simulink model "Trajectory_Tracking_Final"  (R2023b)
settings: Solver=ode1  StartTime=0.0  StopTime=100  FixedStep=SampleTime  MaxStep=0.01  RelTol=1e-3  EnableMultiTasking=on
values from neighbouring files (symbols this model uses):
  Delay = 3    [Prepare_MPC_005.m]
  FilterDer0 = [8.542800360484532896e-02 ... (first row only)    [Prepare_MPC_005.m]
  FilterDer1 = [2.939212680227305530e+00 ... (first row only)    [Prepare_MPC_005.m]
  SampleTime = 0.05    [Prepare_MPC_005.m]
undefined symbols (not defined in the file or in its folder): GetPosition, length_trajectory_s, poly_approx_trajectory, UpdateBoard, xx, yy
libraries: sldrtlib x1
(part 2 of 2)

== system Trajectory_Tracking_Final/Subsystem1/Subsystem/Subsystem5/Subsystem13 ==
  u : Inport
  MATLAB Function11 : MATLAB Function  TreatAsAtomicUnit=on
  MatrixMultiply : Product  Multiplication=Matrix(*)
  Out1 : Outport
  wires:
  [Filter_Coeff_1] -> MatrixMultiply/2
  MATLAB Function11/1(y) -> MatrixMultiply/1
  MatrixMultiply/1 -> Out1/1
  u/1 -> MATLAB Function11/1(u)
  [Initial_MAtrix_Buffer] -> MATLAB Function11/2(Initial_Buffer)

== system Trajectory_Tracking_Final/Subsystem1/Subsystem/Subsystem5/Subsystem14 ==
  u : Inport
  MATLAB Function11 : MATLAB Function  TreatAsAtomicUnit=on
  MatrixMultiply : Product  Multiplication=Matrix(*)
  Out1 : Outport
  wires:
  [Filter_Coeff_1] -> MatrixMultiply/2
  MATLAB Function11/1(y) -> MatrixMultiply/1
  MatrixMultiply/1 -> Out1/1
  u/1 -> MATLAB Function11/1(u)
  [Initial_MAtrix_Buffer] -> MATLAB Function11/2(Initial_Buffer)

== system Trajectory_Tracking_Final/Subsystem1/Subsystem/Subsystem5/Subsystem2 ==
  u : Inport
  MATLAB Function11 : MATLAB Function  TreatAsAtomicUnit=on
  MatrixMultiply : Product  Multiplication=Matrix(*)
  Out1 : Outport
  wires:
  [Filter_Coeff_0] -> MatrixMultiply/2
  MATLAB Function11/1(y) -> MatrixMultiply/1
  MatrixMultiply/1 -> Out1/1
  u/1 -> MATLAB Function11/1(u)
  [Initial_MAtrix_Buffer] -> MATLAB Function11/2(Initial_Buffer)

== system Trajectory_Tracking_Final/Subsystem1/Subsystem/Subsystem5/Subsystem3 ==
  u : Inport
  MATLAB Function11 : MATLAB Function  TreatAsAtomicUnit=on
  MatrixMultiply : Product  Multiplication=Matrix(*)
  Out1 : Outport
  wires:
  [Filter_Coeff_0] -> MatrixMultiply/2
  MATLAB Function11/1(y) -> MatrixMultiply/1
  MatrixMultiply/1 -> Out1/1
  u/1 -> MATLAB Function11/1(u)
  [Initial_MAtrix_Buffer] -> MATLAB Function11/2(Initial_Buffer)

== system Trajectory_Tracking_Final/Subsystem1/Subsystem/Subsystem5/Subsystem4 ==
  u : Inport
  MATLAB Function11 : MATLAB Function  TreatAsAtomicUnit=on
  MatrixMultiply : Product  Multiplication=Matrix(*)
  Out1 : Outport
  wires:
  [Filter_Coeff_0] -> MatrixMultiply/2
  MATLAB Function11/1(y) -> MatrixMultiply/1
  MatrixMultiply/1 -> Out1/1
  u/1 -> MATLAB Function11/1(u)
  [Initial_MAtrix_Buffer] -> MATLAB Function11/2(Initial_Buffer)

== system Trajectory_Tracking_Final/Subsystem1/Subsystem/Subsystem5/Subsystem5 ==
  u : Inport
  Discrete Filter Coefficents : Constant  Value=|
      | [1.574208515729901059e+01
      | 1.586094721714563072e+01
      | -5.994995630757394833e-01
      | -9.191365250349250005e+00
      | -1.170290325508502960e+01
      | -9.922366987693955309e+00
      | -5.638009858585491862e+00
      | -6.380852781707303523e-01
      | 3.289153343139662233e+00
      | 4.355452594936194188e+00
      | 7.725590668082207291e-01
      | -2.327967186368518515e+00]'
  MATLAB Function11 : MATLAB Function  TreatAsAtomicUnit=on
  MatrixMultiply : Product  Multiplication=Matrix(*)
  X_Vel : Outport
  wires:
  Discrete Filter Coefficents/1 -> MatrixMultiply/2
  MATLAB Function11/1(y) -> MatrixMultiply/1
  MatrixMultiply/1 -> X_Vel/1
  u/1 -> MATLAB Function11/1(u)

== system Trajectory_Tracking_Final/Subsystem1/Subsystem/Subsystem5/Subsystem6 ==
  u : Inport
  Discrete Filter Coefficents : Constant  Value=|
      | [1.574208515729901059e+01
      | 1.586094721714563072e+01
      | -5.994995630757394833e-01
      | -9.191365250349250005e+00
      | -1.170290325508502960e+01
      | -9.922366987693955309e+00
      | -5.638009858585491862e+00
      | -6.380852781707303523e-01
      | 3.289153343139662233e+00
      | 4.355452594936194188e+00
      | 7.725590668082207291e-01
      | -2.327967186368518515e+00]'
  MATLAB Function11 : MATLAB Function  TreatAsAtomicUnit=on
  MatrixMultiply : Product  Multiplication=Matrix(*)
  X_Vel1 : Outport
  wires:
  Discrete Filter Coefficents/1 -> MatrixMultiply/2
  MATLAB Function11/1(y) -> MatrixMultiply/1
  MatrixMultiply/1 -> X_Vel1/1
  u/1 -> MATLAB Function11/1(u)

== system Trajectory_Tracking_Final/Subsystem1/Subsystem/Subsystem5/Subsystem7 ==
  u : Inport
  Derivative : Derivative
  Discrete Filter Coefficents : Constant  Value=|
      | [1.574208515729901059e+01
      | 1.586094721714563072e+01
      | -5.994995630757394833e-01
      | -9.191365250349250005e+00
      | -1.170290325508502960e+01
      | -9.922366987693955309e+00
      | -5.638009858585491862e+00
      | -6.380852781707303523e-01
      | 3.289153343139662233e+00
      | 4.355452594936194188e+00
      | 7.725590668082207291e-01
      | -2.327967186368518515e+00]'
  MATLAB Function11 : MATLAB Function  TreatAsAtomicUnit=on
  MatrixMultiply : Product  Multiplication=Matrix(*)
  Scope : Scope  NumInputPorts=2
  Out1 : Outport
  wires:
  Discrete Filter Coefficents/1 -> MatrixMultiply/2
  MATLAB Function11/1(y) -> MatrixMultiply/1
  MatrixMultiply/1 -> Scope/1, Out1/1
  u/1 -> Derivative/1, MATLAB Function11/1(u)
  Derivative/1 -> Scope/2

== system Trajectory_Tracking_Final/Subsystem1/Subsystem/Subsystem5/Subsystem8 ==
  u : Inport
  Discrete Filter Coefficents : Constant  Value=|
      | [1.574208515729901059e+01
      | 1.586094721714563072e+01
      | -5.994995630757394833e-01
      | -9.191365250349250005e+00
      | -1.170290325508502960e+01
      | -9.922366987693955309e+00
      | -5.638009858585491862e+00
      | -6.380852781707303523e-01
      | 3.289153343139662233e+00
      | 4.355452594936194188e+00
      | 7.725590668082207291e-01
      | -2.327967186368518515e+00]'
  MATLAB Function11 : MATLAB Function  TreatAsAtomicUnit=on
  MatrixMultiply : Product  Multiplication=Matrix(*)
  Out1 : Outport
  wires:
  Discrete Filter Coefficents/1 -> MatrixMultiply/2
  MATLAB Function11/1(y) -> MatrixMultiply/1
  MatrixMultiply/1 -> Out1/1
  u/1 -> MATLAB Function11/1(u)

== system Trajectory_Tracking_Final/Subsystem1/Subsystem/Subsystem5/Subsystem9 ==
  u : Inport
  Derivative : Derivative
  Discrete Filter Coefficents : Constant  Value=|
      | [1.574208515729901059e+01
      | 1.586094721714563072e+01
      | -5.994995630757394833e-01
      | -9.191365250349250005e+00
      | -1.170290325508502960e+01
      | -9.922366987693955309e+00
      | -5.638009858585491862e+00
      | -6.380852781707303523e-01
      | 3.289153343139662233e+00
      | 4.355452594936194188e+00
      | 7.725590668082207291e-01
      | -2.327967186368518515e+00]'
  MATLAB Function11 : MATLAB Function  TreatAsAtomicUnit=on
  MatrixMultiply : Product  Multiplication=Matrix(*)
  Scope : Scope  NumInputPorts=2
  Out1 : Outport
  wires:
  Discrete Filter Coefficents/1 -> MatrixMultiply/2
  MATLAB Function11/1(y) -> MatrixMultiply/1
  Derivative/1 -> Scope/2
  u/1 -> Derivative/1, MATLAB Function11/1(u)
  MatrixMultiply/1 -> Scope/1, Out1/1

== matlab function Trajectory_Tracking_Final/Subsystem1/Subsystem/Subsystem5/MATLAB Function ==
  data: Initial_MAtrix output
function Initial_MAtrix = Immutable_Constant_Matrix()

Initial_MAtrix = ones(10,1);

== matlab function Trajectory_Tracking_Final/Subsystem1/Subsystem/Limit Input/MATLAB Function5 ==
  data: PWL input; PWL_Limit output; Position input; epsilon input
function PWL_Limit = fcn(PWL,Position,epsilon)

if (PWL < 0) && (Position-epsilon <= 0)
 PWL_Limit = 0;
else if (PWL > 0) && (Position+epsilon >= 0.49876)
     PWL_Limit = 0    ;
else
 PWL_Limit = PWL;
end
end

== matlab function Trajectory_Tracking_Final/Subsystem1/Subsystem/Limit Input/MATLAB Function6 ==
  data: PWL input; PWL_Limit output; Position input; epsilon input

function PWL_Limit = fcn(PWL,Position,epsilon)

if (PWL < 0) && (Position-epsilon <= 0)
 PWL_Limit = 0;
else if (PWL > 0) && (Position+epsilon >= 0.62159)
     PWL_Limit = 0    ;
else
 PWL_Limit = PWL;
end
end

== matlab function Trajectory_Tracking_Final/SOLVE OCP /Subsystem/Delete L ==
  data: x10 input; x_8 output
function x_8 = fcn(x10)
relevantstates = [1,2,4,5,6,7,9,10];
x_8 =x10(relevantstates);

== matlab function Trajectory_Tracking_Final/SOLVE OCP /Subsystem5/MPC 1/MATLAB Function ==
  data: x input; x_warm output
function x_warm = fcn(x)
x_warm = [x(:,3:end) x(:,end)];

== matlab function Trajectory_Tracking_Final/Subsystem1/Subsystem/Limit Input/MATLAB Function4 ==
  data: PWL input; PWL_Limit output; Position input; epsilon input
function PWL_Limit = fcn(PWL,Position,epsilon)

if (PWL < 0) && (Position-epsilon <= 0)
 PWL_Limit = 0;
else if (PWL > 0) && (Position+epsilon >= 0.55004)
     PWL_Limit = 0    ;
else
 PWL_Limit = PWL;
end
end
% 0.55004

== matlab function Trajectory_Tracking_Final/Subsystem1/Subsystem/Subsystem5/Subsystem/MATLAB Function11 ==
  settings: updateMethod=DISCRETE
  data: u input; y output size=[1,N_Coeff]; Initial_Buffer input
function y = CircularBuffer(u,Initial_Buffer)
%#codegen
% Function to implement a simple N element circular buffer

% Define the internal buffer variable as persistent
persistent buffer



% Initialize the buffer the first time through
if isempty(buffer)
    % Initialize the buffer
    buffer = Initial_Buffer*u;
    % buff_entrys = 1;
    buffer(1) = u;
else
    % wenn nicht leer, dann schiebe eins hoch 
    buff2 = buffer; 
    buffer = [u; buff2(1:end-1)];
end

% Output the buffer
y = buffer';

end

== matlab function Trajectory_Tracking_Final/SOLVE OCP /Subsystem5/MPC 1/MATLAB Function1 ==
  data: lam_g input; lam_g_warm output
function lam_g_warm = fcn(lam_g)
lam_g_warm = lam_g;

== matlab function Trajectory_Tracking_Final/SOLVE OCP /Subsystem5/MPC 1/MATLAB Function2 ==
  data: u input; u_warm output size=DimU
function u_warm = fcn(u)

u_warm = [u(:,2:end) u(:,end)];

== matlab function Trajectory_Tracking_Final/SOLVE OCP /Subsystem5/MATLAB Function3 ==
  data: u input; u_plant output size=[1,1]; x input; x_new output
function [u_plant,x_new] = fcn(u,x)

x_new = x(:,2);
u_plant = u(:,1);

== matlab function Trajectory_Tracking_Final/Nonlinear Model/MATLAB Function4 ==
  data: x_in input; PWM input; x_end output; SampleTime input
function x_end   = Integrate_rk4(x_in, PWM,SampleTime)

% X_PWM_Simtime = PWM(1,:);
% Y_PWM_Simtime = PWM(2,:);
% Z_PWM_Simtime = PWM(3,:);
dt =  0.0002; % Time step for RK4 integration
% nSteps = 451;
nSteps = SampleTime/dt +1;
% l0 = 0.1712;
params = struct;
% Initialize output matrix for the RK4 results
% Apply coordinate transform to fit model
% x = [x_in(1) x_in(2) x_in(3)+l0  x_in(4) x_in(5) x_in(6) (x_in(7)) x_in(8) x_in(9) x_in(10)]; % Initial state
x = x_in';
% rk4Results = zeros(nSteps, length(x));
% rk4Results(1, :) = x_in'; % Initial state

for i = 1:nSteps-1
    % Current input
    u = [PWM(1) PWM(2) 0];
    % RK4 Integration
    k1 = crane3DModel_derivation(x, u);
    k2 = crane3DModel_derivation(x + 0.5*dt*k1, u);
    k3 = crane3DModel_derivation(x + 0.5*dt*k2, u);
    k4 = crane3DModel_derivation(x + dt*k3, u);
    
    x = x + dt*(k1 + 2*k2 + 2*k3 + k4)/6;
    % rk4Results(i+1, :) = [x(1), x(2), x(3)-l0,(x(4)), x(5) ,x(6), x(7), x(8), x(9), x(10)];
  % rk4Results(i+1, :) = x;

end
x_end = x;
end

== matlab function Trajectory_Tracking_Final/Subsystem1/Subsystem/Subsystem5/Subsystem5/MATLAB Function11 ==
  settings: updateMethod=DISCRETE  sampleTime=0.01
  data: u input; y output size=1
function y = CircularBuffer(u)
%#codegen
% Function to implement a simple N element circular buffer

% Define the internal buffer variable as persistent
persistent buffer

N = 12;

% Initialize the buffer the first time through
if isempty(buffer)
    % Initialize the buffer
    buffer = zeros(N,1);
    % buff_entrys = 1;
    buffer(1) = u;
else
    % wenn nicht leer, dann schiebe eins hoch 
    buff2 = buffer; 
    buffer = [u; buff2(1:N-1)];
end

% Output the buffer
y = buffer';

end

== matlab function Trajectory_Tracking_Final/Subsystem1/Subsystem/Subsystem5/Subsystem6/MATLAB Function11 ==
  settings: updateMethod=DISCRETE  sampleTime=0.01
  data: u input; y output
function y = CircularBuffer(u)
%#codegen
% Function to implement a simple N element circular buffer

% Define the internal buffer variable as persistent
persistent buffer

N = 12;

% Initialize the buffer the first time through
if isempty(buffer)
    % Initialize the buffer
    buffer = zeros(N,1);
    % buff_entrys = 1;
    buffer(1) = u;
else
    % wenn nicht leer, dann schiebe eins hoch 
    buff2 = buffer; 
    buffer = [u; buff2(1:N-1)];
end

% Output the buffer
y = buffer';

end

== matlab function Trajectory_Tracking_Final/Subsystem1/Subsystem/Subsystem5/Subsystem7/MATLAB Function11 ==
  settings: updateMethod=DISCRETE  sampleTime=0.01
  data: u input; y output
function y = CircularBuffer(u)
%#codegen
% Function to implement a simple N element circular buffer

% Define the internal buffer variable as persistent
persistent buffer

N = 12;

% Initialize the buffer the first time through
if isempty(buffer)
    % Initialize the buffer
    buffer = zeros(N,1);
    % buff_entrys = 1;
    buffer(1) = u;
else
    % wenn nicht leer, dann schiebe eins hoch 
    buff2 = buffer; 
    buffer = [u; buff2(1:N-1)];
end

% Output the buffer
y = buffer';

end

== matlab function Trajectory_Tracking_Final/Subsystem1/Subsystem/Subsystem5/Subsystem8/MATLAB Function11 ==
  settings: updateMethod=DISCRETE  sampleTime=0.01
  data: u input; y output
function y = CircularBuffer(u)
%#codegen
% Function to implement a simple N element circular buffer

% Define the internal buffer variable as persistent
persistent buffer

N = 12;

% Initialize the buffer the first time through
if isempty(buffer)
    % Initialize the buffer
    buffer = zeros(N,1);
    % buff_entrys = 1;
    buffer(1) = u;
else
    % wenn nicht leer, dann schiebe eins hoch 
    buff2 = buffer; 
    buffer = [u; buff2(1:N-1)];
end

% Output the buffer
y = buffer';

end

== matlab function Trajectory_Tracking_Final/Subsystem1/Subsystem/Subsystem5/Subsystem9/MATLAB Function11 ==
  settings: updateMethod=DISCRETE  sampleTime=0.01
  data: u input; y output
function y = CircularBuffer(u)
%#codegen
% Function to implement a simple N element circular buffer

% Define the internal buffer variable as persistent
persistent buffer

N = 12;

% Initialize the buffer the first time through
if isempty(buffer)
    % Initialize the buffer
    buffer = zeros(N,1);
    % buff_entrys = 1;
    buffer(1) = u;
else
    % wenn nicht leer, dann schiebe eins hoch 
    buff2 = buffer; 
    buffer = [u; buff2(1:N-1)];
end

% Output the buffer
y = buffer';

end

== matlab function Trajectory_Tracking_Final/Subsystem3/dry_friction_compensation ==
  data: x input; u input; u_compensated output
function u_compensated = fcn(x,u)
% u_compensated = u+[-0.1576*sign(100*x(5)); -0.1232*sign(100*x(6))];
% u_compensated = u+[-0.1576*sign(100*u(1)); -0.1232*sign(100*u(2))];
u_compensated = zeros(2,1);
if abs(u(1)) > 0.01
u_compensated(1) = u(1) +  0.1576*tanh(200*x(6));
% u_compensated(1) = u(1) +  0.006*tanh(200*x(6));
end
if abs(u(2)) > 0.01
u_compensated(2) = u(2) +  0.1232*tanh(200*x(7));
end
% u_compensated = u + [0.1576*tanh(2000*x(6)); 0.1232*tanh(2000*x(7))];

== matlab function Trajectory_Tracking_Final/Nonlinear Model/MATLAB Function3 ==
  data: x input; current output
function current = fcn(x)
current = [x(:,1)];

== matlab function Trajectory_Tracking_Final/Subsystem1/Subsystem/MATLAB Function ==
  data: Positions output size=[1, 5]; PWM_X input; PWM_Y input; PWM_Z input; Time output
function [Positions,Time]  = Driver(PWM_X, PWM_Y, PWM_Z)

persistent starttime


% Input = [0.1 0.1 0.1];
Positions = [0 0 0 0 0];
PWM = [0 0 0];
Time1 = 0;
[Positions Time1] = UpdateBoard([PWM_X, PWM_Y, PWM_Z]);
if isempty(starttime)
    starttime = Time1;
end
Time = (Time1 - starttime)/1000;

% Positions = [0,0,0,0,0];
% % Positions = getEncoderCounter();
% Positions = Positions';
end

== matlab function Trajectory_Tracking_Final/SOLVE OCP /Nonlinear Model1/MATLAB Function ==
  data: x input; x_bound output
function x_bound = fcn(x)
x_bound = x;
if x_bound(1) < 0.01
    x_bound(1) = 0.01;
end
if x_bound(1) > 0.49
    x_bound(1) = 0.49;
end
if x_bound(2) < 0.01
    x_bound(2) = 0.01;
end
if x_bound(2) > 0.59
    x_bound(2) = 0.59;
end

== matlab function Trajectory_Tracking_Final/SOLVE OCP /Subsystem4/MATLAB Function3 ==
  data: u input; u_plant output size=[1,1]; x input
function u_plant = fcn(u,x)

x_new = x(:,2);
u_plant = u(:,1);

== matlab function Trajectory_Tracking_Final/SOLVE OCP /Subsystem5/MPC 1/Subsystem4/MATLAB Function8 ==
  data: traj input; first_elemt_traj output
function first_elemt_traj = getfirstelement(traj)

first_elemt_traj = traj(:,1);

== matlab function Trajectory_Tracking_Final/SOLVE OCP /Subsystem4/MPC 1/MATLAB Function ==
  data: x input; x_warm output
function x_warm = fcn(x)
x_warm = [x(:,3:end) x(:,end)];

== matlab function Trajectory_Tracking_Final/SOLVE OCP /Subsystem/MATLAB Function10 ==
  data: x_18 input; x_X output; x_Y output
function [x_X,x_Y] = add_int(x_18)
x_X = zeros(4,1);
x_Y = zeros(4,1);
x_X(1) = x_18(1);
x_Y(1) = x_18(2);
x_X(2) = x_18(3);
x_Y(2) = x_18(4);
x_X(3) = x_18(5);
x_Y(3) = x_18(6);
x_X(4) = x_18(7);
x_Y(4) = x_18(8);

== matlab function Trajectory_Tracking_Final/SOLVE OCP /Subsystem4/MPC 1/MATLAB Function1 ==
  data: lam_g input; lam_g_warm output
function lam_g_warm = fcn(lam_g)
lam_g_warm = lam_g;

== matlab function Trajectory_Tracking_Final/SOLVE OCP /Nonlinear Model1/MATLAB Function4 ==
  data: x_in input; PWM input; x_end output; SampleTime input; Delay input
function x_end = Integrate_rk4(x_in, PWM,SampleTime,Delay)

% X_PWM_Simtime = PWM(1,:);
% Y_PWM_Simtime = PWM(2,:);
% Z_PWM_Simtime = PWM(3,:);
dt =  0.001; % Time step for RK4 integration
% nSteps = 451;
nSteps = Delay*(SampleTime/dt) +1;
Delay = ceil(Delay);
time_full = [0:dt:nSteps*dt-dt];
time_red = [0:SampleTime:Delay*SampleTime];
Signal = PWM(:,Delay+1:-1:1)
Signal_interp1 = interp1(time_red, Signal(1,:), time_full, 'previous');  % You can change 'linear' to other methods like 'spline', 'pchip', etc.
Signal_interp2 = interp1(time_red, Signal(2,:), time_full, 'previous');  % You can change 'linear' to other methods like 'spline', 'pchip', etc.

% l0 = 0.1712;
params = struct;
% Initialize output matrix for the RK4 results
% Apply coordinate transform to fit model
% x = [x_in(1) x_in(2) x_in(3)+l0  x_in(4) x_in(5) x_in(6) (x_in(7)) x_in(8) x_in(9) x_in(10)]; % Initial state
x = x_in';
% rk4Results = zeros(nSteps, length(x));
% rk4Results(1, :) = x_in'; % Initial state

for i = 1:nSteps-1
    % Current input
    u = [Signal_interp1(:,i) Signal_interp2(:,i) 0];
    % RK4 Integration
    k1 = crane3DModel_derivation(x, u);
    k2 = crane3DModel_derivation(x + 0.5*dt*k1, u);
    k3 = crane3DModel_derivation(x + 0.5*dt*k2, u);
    k4 = crane3DModel_derivation(x + dt*k3, u);
    
    x = x + dt*(k1 + 2*k2 + 2*k3 + k4)/6;
    % rk4Results(i+1, :) = [x(1), x(2), x(3)-l0,(x(4)), x(5) ,x(6), x(7), x(8), x(9), x(10)];
  % rk4Results(i+1, :) = x;

end
x_end = x;
end

== matlab function Trajectory_Tracking_Final/SOLVE OCP /Nonlinear Model1/MATLAB Function11 ==
  settings: updateMethod=DISCRETE
  data: u input; y output size=[3,7]
function y = CircularBuffer(u)
%#codegen
% Function to implement a simple N element circular buffer

% Define the internal buffer variable as persistent
persistent buffer
Initial_Buffer = ones(3, 7);

% Initialize the buffer the first time through
if isempty(buffer)
    % Initialize the buffer with the initial buffer
    buffer = zeros(3, 7);
    % Place the first input into the buffer
    buffer(:,1) = u;
else
    % Shift the buffer and insert the new input at the beginning
    buffer = [u, buffer(:,1:end-1)];
end

% Output the buffer
y = buffer;

end

== matlab function Trajectory_Tracking_Final/SOLVE OCP /Subsystem5/MPC 1/MATLAB Function3 ==
  data: x input; current output
function current = fcn(x)
current = [x(:,1)];

== matlab function Trajectory_Tracking_Final/SOLVE OCP /Subsystem4/MPC 1/MATLAB Function2 ==
  data: u input; u_warm output size=DimU
function u_warm = fcn(u)

u_warm = [u(:,2:end) u(:,end)];

== matlab function Trajectory_Tracking_Final/SOLVE OCP /Subsystem4/MPC 1/MATLAB Function3 ==
  data: x input; current output
function current = fcn(x)
current = [x(:,1)];

== matlab function Trajectory_Tracking_Final/SOLVE OCP /Subsystem4/MPC 1/Subsystem4/MATLAB Function8 ==
  data: traj input; first_elemt_traj output
function first_elemt_traj = getfirstelement(traj)

first_elemt_traj = traj(:,1);

== matlab function Trajectory_Tracking_Final/TRajcetory from design reference1/Scenario1/MATLAB Function11 ==
  data: traj input; lin_traj output
function lin_traj = linearize_trajectory(traj)
lin_traj = zeros(2,2);
lin_traj(:,1) = traj(1:2,1);
lin_traj(:,2) = traj(1:2,end);
end

== matlab function Trajectory_Tracking_Final/TRajcetory from design reference1/Scenario1/MATLAB Function5 ==
  data: t input; y output; timestep input; Delay input; y_ output
function [y,y_]  = trajectory(t,timestep,Delay)
l = 21;

y = zeros(4,l);
y_diff = zeros(2,l);
y_order_0 = zeros(2,l);
origin = [0.3 ; 0.3];
radius = 0.18;
f =3;
for i = 1:l
    y_order_0(:,i) = [origin(1)+ radius*sin(f*(t+i*timestep));origin(2)+radius*cos(f*(t+i*timestep))];
    y_diff(:,i) =  [radius*f*cos(f*(t+i*timestep));-radius*f*sin(f*(t+i*timestep))];
end
y = [y_order_0 ;y_diff];

t_ = t-Delay*timestep;
y_ = zeros(4,l);
y_diff = zeros(2,l);
y_order_0 = zeros(2,l);
origin = [0.3 ; 0.3];
radius = 0.2;

for i = 1:l
    y_order_0(:,i) = [origin(1)+ radius*sin(f*(t+i*timestep));origin(2)+radius*cos(f*(t+i*timestep))];
    y_diff(:,i) =  [radius*f*cos(f*(t+i*timestep));-radius*f*sin(f*(t+i*timestep))];
end
y_ = [y_order_0 ;y_diff];

== matlab function Trajectory_Tracking_Final/Subsystem1/Subsystem/Subsystem5/Subsystem1/MATLAB Function11 ==
  settings: updateMethod=DISCRETE
  data: u input; y output size=[1,N_Coeff]; Initial_Buffer input
function y = CircularBuffer(u,Initial_Buffer)
%#codegen
% Function to implement a simple N element circular buffer

% Define the internal buffer variable as persistent
persistent buffer



% Initialize the buffer the first time through
if isempty(buffer)
    % Initialize the buffer
    buffer = Initial_Buffer*u;
    % buff_entrys = 1;
    buffer(1) = u;
else
    % wenn nicht leer, dann schiebe eins hoch 
    buff2 = buffer; 
    buffer = [u; buff2(1:end-1)];
end

% Output the buffer
y = buffer';

end

== matlab function Trajectory_Tracking_Final/TRajcetory from design reference/Subsystem5/Delete L ==
  data: x10 input; x_8 output
function x_8 = fcn(x10)
relevantstates = [1,2,4,5,6,7,9,10];
x_8 =x10(relevantstates);

== matlab function Trajectory_Tracking_Final/TRajcetory from design reference/Subsystem5/MATLAB Function ==
  data: x input; x_warm output
function x_warm = fcn(x)
x_warm = [x(:,3:end) x(:,end)];

== matlab function Trajectory_Tracking_Final/TRajcetory from design reference/Subsystem5/MATLAB Function1 ==
  data: lam_g input; lam_g_warm output
function lam_g_warm = fcn(lam_g)
lam_g_warm = lam_g;

== matlab function Trajectory_Tracking_Final/TRajcetory from design reference/Subsystem5/MATLAB Function10 ==
  data: x_18 input; x_out output; x_9 input
function x_out = add_int(x_18,x_9)
x_out = zeros(10,1);
x_out(1) = x_18(1);
x_out(2) = x_18(2);
x_out(3) = x_18(3);
x_out(4) = x_18(4);
x_out(5) = x_18(5);
x_out(6) = x_18(6);
x_out(7) = x_18(7);
x_out(8) = x_18(8);
x_out(9) = x_9(9);
x_out(10) = x_9(10);
% x_out(11) = x_9(11);
% x_out(12) = x_9(12);

if x_out(1) < 0 
    x_out(1) = 0;
end
if x_out(2) < 0 
    x_out(2) = 0;
end

== matlab function Trajectory_Tracking_Final/TRajcetory from design reference/Subsystem5/MATLAB Function2 ==
  data: u input; u_warm output size=DimU; Delay input
function u_warm = fcn(u,Delay)
Delay = 3;
u_warm = [u(:,(Delay+1):end) u(:,end)];

== matlab function Trajectory_Tracking_Final/TRajcetory from design reference/Subsystem5/MATLAB Function3 ==
  data: u input; u_new output size=[2,Delay]; u_plant output size=[2,1]; x input; x_new output; Delay input
function [u_new,u_plant,x_new] = fcn(u,x,Delay)
% size(u)
% size(x)
Delay = 3;
u_new = zeros(2,Delay);
u_new = u(:,1:Delay);
x_new = x(:,2);
u_plant = u(:,Delay+1);

== matlab function Trajectory_Tracking_Final/TRajcetory from design reference/Subsystem5/Subsystem4/MATLAB Function8 ==
  data: traj input; first_elemt_traj output
function first_elemt_traj = getfirstelement(traj)

first_elemt_traj = traj(:,1);

== matlab function Trajectory_Tracking_Final/TRajcetory from design reference1/Subsystem1/MATLAB Function6 ==
  data: x input; Payload_x output; Payload_y output; Payload_x_der output; Payload_y_der output
function [Payload_x,Payload_y,Payload_x_der,Payload_y_der] = PAyload_calc(x)
Payload_x = x(1)+ 0.5478*x(4);
 Payload_y = x(2)+ 0.5478*x(5);
 Payload_x_der = x(6)+ 0.5478*x(9);
 Payload_y_der = x(7)+ 0.5478*x(10);

== matlab function Trajectory_Tracking_Final/TRajcetory from design reference1/Subsystem1/MATLAB Function7 ==
  data: traj input; first_elemt_traj output
function first_elemt_traj = getfirstelement(traj)

first_elemt_traj = traj(:,1);

== matlab function Trajectory_Tracking_Final/Subsystem1/Subsystem/Subsystem5/Subsystem2/MATLAB Function11 ==
  settings: updateMethod=DISCRETE
  data: u input; y output size=[1,N_Coeff]; Initial_Buffer input
function y = CircularBuffer(u,Initial_Buffer)
%#codegen
% Function to implement a simple N element circular buffer

% Define the internal buffer variable as persistent
persistent buffer



% Initialize the buffer the first time through
if isempty(buffer)
    % Initialize the buffer
    buffer = Initial_Buffer*u;
    % buff_entrys = 1;
    buffer(1) = u;
else
    % wenn nicht leer, dann schiebe eins hoch 
    buff2 = buffer; 
    buffer = [u; buff2(1:end-1)];
end

% Output the buffer
y = buffer';

end

== matlab function Trajectory_Tracking_Final/SOLVE OCP /Subsystem5/MPC 1/MATLAB Function4 ==
  data: u input; y output
function y = fcn(u)

y = u(1,1);

== matlab function Trajectory_Tracking_Final/SOLVE OCP /Subsystem5/MPC 1/MATLAB Function5 ==
  data: x input; current output
function current = fcn(x)
current = [x(:,1)];

== matlab function Trajectory_Tracking_Final/SOLVE OCP /Subsystem5/Trajectroy ==
  data: coeffs input; evaluated_polynomials_X output; t input size=[1 1]
function evaluated_polynomials_X = evaluatePolynomials(coeffs, t)


    % % Initialize an array to hold the evaluated polynomials
    num_trajectories = size(coeffs, 1); % Number of trajectories (rows of coeffs)
    % evaluated_polynomials = casadi.MX(num_trajectories, 1);
     evaluated_polynomials = zeros(num_trajectories, 1);
    % 
    % Loop over each set of coefficients (each trajectory)
    for j = 1:num_trajectories
        % Get the coefficients for this trajectory
        current_coeffs = coeffs(j, :);
        % Find the degree of the polynomial based on the number of coefficients
        degree = length(current_coeffs) - 1;

        % Initialize the polynomial expression to zero for this trajectory
        % current_polynomial = casadi.MX(1,1);
        current_polynomial = zeros(1,1);
        % Evaluate the polynomial using a loop, considering the order of coefficients
        for i = 0:degree
            % Add each term of the polynomial
            current_polynomial = current_polynomial + current_coeffs(degree + 1 - i) * t^i;
        end

        % Evaluate the current polynomial at the given time t
        evaluated_polynomials(j) = (current_polynomial);
    end
    if num_trajectories ==8
    % evaluated_polynomials(1) = 0.25 + 0.2*sin(t);
    % evaluated_polynomials(2) = 0.25 + 0.2*cos(t);
    % evaluated_polynomials(3) = 0;
    % evaluated_polynomials(3:8) = zeros(6,1);
    else
        % evaluated_polynomials = zeros(2,1);
    end
    evaluated_polynomials_X = evaluated_polynomials([1,3,5,7]);
end

== matlab function Trajectory_Tracking_Final/SOLVE OCP /Subsystem1/MATLAB Function3 ==
  data: u input; u_plant output size=[1,1]; x input; x_new output
function [u_plant,x_new] = fcn(u,x)

x_new = x(:,2);
u_plant = u(:,1);

== matlab function Trajectory_Tracking_Final/SOLVE OCP /Subsystem1/MPC 1/MATLAB Function ==
  data: x input; x_warm output
function x_warm = fcn(x)
x_warm = [x(:,3:end) x(:,end)];

== matlab function Trajectory_Tracking_Final/SOLVE OCP /Subsystem1/MPC 1/MATLAB Function1 ==
  data: lam_g input; lam_g_warm output
function lam_g_warm = fcn(lam_g)
lam_g_warm = lam_g;

== matlab function Trajectory_Tracking_Final/SOLVE OCP /Subsystem1/MPC 1/MATLAB Function2 ==
  data: u input; u_warm output size=DimU
function u_warm = fcn(u)

u_warm = [u(:,2:end) u(:,end)];

== matlab function Trajectory_Tracking_Final/SOLVE OCP /Subsystem1/MPC 1/MATLAB Function3 ==
  data: x input; current output
function current = fcn(x)
current = [x(:,1)];

== matlab function Trajectory_Tracking_Final/SOLVE OCP /Subsystem1/MPC 1/MATLAB Function4 ==
  data: u input; y output
function y = fcn(u)

y = u(1,1);

== matlab function Trajectory_Tracking_Final/SOLVE OCP /Subsystem1/MPC 1/MATLAB Function5 ==
  data: x input; current output
function current = fcn(x)
current = [x(:,1)];

== matlab function Trajectory_Tracking_Final/SOLVE OCP /Subsystem1/MPC 1/Subsystem4/MATLAB Function8 ==
  data: traj input; first_elemt_traj output
function first_elemt_traj = getfirstelement(traj)

first_elemt_traj = traj(:,1);

== matlab function Trajectory_Tracking_Final/Subsystem1/Subsystem/Subsystem5/Subsystem3/MATLAB Function11 ==
  settings: updateMethod=DISCRETE
  data: u input; y output size=[1,N_Coeff]; Initial_Buffer input
function y = CircularBuffer(u,Initial_Buffer)
%#codegen
% Function to implement a simple N element circular buffer

% Define the internal buffer variable as persistent
persistent buffer



% Initialize the buffer the first time through
if isempty(buffer)
    % Initialize the buffer
    buffer = Initial_Buffer*u;
    % buff_entrys = 1;
    buffer(1) = u;
else
    % wenn nicht leer, dann schiebe eins hoch 
    buff2 = buffer; 
    buffer = [u; buff2(1:end-1)];
end

% Output the buffer
y = buffer';

end

== matlab function Trajectory_Tracking_Final/SOLVE OCP /Subsystem1/Trajectroy ==
  data: coeffs input; evaluated_polynomials_X output; t input size=[1 1]
function evaluated_polynomials_X = evaluatePolynomials(coeffs, t)


    % % Initialize an array to hold the evaluated polynomials
    num_trajectories = size(coeffs, 1); % Number of trajectories (rows of coeffs)
    % evaluated_polynomials = casadi.MX(num_trajectories, 1);
     evaluated_polynomials = zeros(num_trajectories, 1);
    % 
    % Loop over each set of coefficients (each trajectory)
    for j = 1:num_trajectories
        % Get the coefficients for this trajectory
        current_coeffs = coeffs(j, :);
        % Find the degree of the polynomial based on the number of coefficients
        degree = length(current_coeffs) - 1;

        % Initialize the polynomial expression to zero for this trajectory
        % current_polynomial = casadi.MX(1,1);
        current_polynomial = zeros(1,1);
        % Evaluate the polynomial using a loop, considering the order of coefficients
        for i = 0:degree
            % Add each term of the polynomial
            current_polynomial = current_polynomial + current_coeffs(degree + 1 - i) * t^i;
        end

        % Evaluate the current polynomial at the given time t
        evaluated_polynomials(j) = (current_polynomial);
    end
    if num_trajectories ==8
    % evaluated_polynomials(1) = 0.25 + 0.2*sin(t);
    % evaluated_polynomials(2) = 0.25 + 0.2*cos(t);
    % evaluated_polynomials(3) = 0;
    % evaluated_polynomials(3:8) = zeros(6,1);
    else
        % evaluated_polynomials = zeros(2,1);
    end
    evaluated_polynomials_X = evaluated_polynomials([1,3,5,7]);
end

== matlab function Trajectory_Tracking_Final/MATLAB Function ==
  data: u input; u output; t input; enable input
function u  = disturbance(u, t,enable)
if ~enable
u = u;
else
    % Define the time intervals for disturbances
    Time_Disturbance1 = [20, 23];
    Time_Disturbance2 = [40, 41];
    Time_Disturbance3 = [58, 60];
    Time_Disturbance4 = [80, 90];

    % Determine which disturbance interval t falls into
    if t >= min(Time_Disturbance1) && t <= max(Time_Disturbance1)
        current_Disturbance = 'Time_Disturbance1';
    elseif t >= min(Time_Disturbance2) && t <= max(Time_Disturbance2)
        current_Disturbance = 'Time_Disturbance2';
    elseif t >= min(Time_Disturbance3) && t <= max(Time_Disturbance3)
        current_Disturbance = 'Time_Disturbance3';
    elseif t >= min(Time_Disturbance4) && t <= max(Time_Disturbance4)
        current_Disturbance = 'Time_Disturbance4';
    else
        current_Disturbance = 'None';
    end

    % Switch statement based on the current disturbance
    switch current_Disturbance
        case 'Time_Disturbance1'

        u = ones(2,1);
        case 'Time_Disturbance2'

            u = zeros(2,1);


        case 'Time_Disturbance3'
u(1) = -1*sin(3*t);
u(2) = 0 ;
        case 'Time_Disturbance4'
       u(1) = u(1) + 0.4*sin(4*t);
u(2) = u(2) + 0.4*sin(5*t); 
        otherwise

    end
end
end

== matlab function Trajectory_Tracking_Final/SOLVE OCP /Subsystem2/Delete L ==
  data: x10 input; x_8 output
function x_8 = fcn(x10)
relevantstates = [1,2,4,5,6,7,9,10];
x_8 =x10(relevantstates);

== matlab function Trajectory_Tracking_Final/SOLVE OCP /Subsystem2/MATLAB Function10 ==
  data: x_18 input; x_X output; x_Y output
function [x_X,x_Y] = add_int(x_18)
x_X = zeros(4,1);
x_Y = zeros(4,1);
x_X(1) = x_18(1);
x_Y(1) = x_18(2);
x_X(2) = x_18(3);
x_Y(2) = x_18(4);
x_X(3) = x_18(5);
x_Y(3) = x_18(6);
x_X(4) = x_18(7);
x_Y(4) = x_18(8);

== matlab function Trajectory_Tracking_Final/TRajcetory from design reference/Scenario1/MATLAB Function11 ==
  data: traj input; lin_traj output
function lin_traj = linearize_trajectory(traj)
lin_traj = zeros(2,2);
lin_traj(:,1) = traj(1:2,1);
lin_traj(:,2) = traj(1:2,end);
end

== matlab function Trajectory_Tracking_Final/TRajcetory from design reference/Scenario1/MATLAB Function5 ==
  data: t input; y output; timestep input; Delay input; y_ output
function [y,y_]  = trajectory(t,timestep,Delay)
l = 21;

y = zeros(4,l);
y_diff = zeros(2,l);
y_order_0 = zeros(2,l);
origin = [0.3 ; 0.3];
radius = 0.3;
% f =3.5;
f = 3.5;
for i = 1:l
    y_order_0(:,i) = [origin(1)+ radius*sin(f*(t+i*timestep));origin(2)+radius*cos(f*(t+i*timestep))];
    y_diff(:,i) =  [radius*f*cos(f*(t+i*timestep));-radius*f*sin(f*(t+i*timestep))];
end
y = [y_order_0 ;y_diff];

t_ = t-Delay*timestep;
y_ = zeros(4,l);
y_diff = zeros(2,l);
y_order_0 = zeros(2,l);
origin = [0.3 ; 0.3];
radius = 0.2;

for i = 1:l
    y_order_0(:,i) = [origin(1)+ radius*sin(f*(t+i*timestep));origin(2)+radius*cos(f*(t+i*timestep))];
    y_diff(:,i) =  [radius*f*cos(f*(t+i*timestep));-radius*f*sin(f*(t+i*timestep))];
end
y_ = [y_order_0 ;y_diff];

== matlab function Trajectory_Tracking_Final/TRajcetory from design reference/Subsystem1/MATLAB Function6 ==
  data: x input; Payload_x output; Payload_y output; Payload_x_der output; Payload_y_der output
function [Payload_x,Payload_y,Payload_x_der,Payload_y_der] = PAyload_calc(x)
Payload_x = x(1)+ 0.5478*x(4);
 Payload_y = x(2)+ 0.5478*x(5);
 Payload_x_der = x(6)+ 0.5478*x(9);
 Payload_y_der = x(7)+ 0.5478*x(10);

== matlab function Trajectory_Tracking_Final/TRajcetory from design reference/Subsystem1/MATLAB Function7 ==
  data: traj input; first_elemt_traj output
function first_elemt_traj = getfirstelement(traj)

first_elemt_traj = traj(:,1);

== matlab function Trajectory_Tracking_Final/TRajcetory from design reference1/Subsystem2/MATLAB Function11 ==
  data: traj input; lin_traj output
function lin_traj = linearize_trajectory(traj)
lin_traj = zeros(2,2);
lin_traj(:,1) = traj(1:2,1);
lin_traj(:,2) = traj(1:2,end);
end

== matlab function Trajectory_Tracking_Final/TRajcetory from design reference/Subsystem2/MATLAB Function11 ==
  data: traj input; lin_traj output
function lin_traj = linearize_trajectory(traj)
lin_traj = zeros(2,2);
lin_traj(:,1) = traj(1:2,1);
lin_traj(:,2) = traj(1:2,end);
end

== matlab function Trajectory_Tracking_Final/Subsystem1/Subsystem/Subsystem5/Subsystem4/MATLAB Function11 ==
  settings: updateMethod=DISCRETE
  data: u input; y output size=[1,N_Coeff]; Initial_Buffer input
function y = CircularBuffer(u,Initial_Buffer)
%#codegen
% Function to implement a simple N element circular buffer

% Define the internal buffer variable as persistent
persistent buffer



% Initialize the buffer the first time through
if isempty(buffer)
    % Initialize the buffer
    buffer = Initial_Buffer*u;
    % buff_entrys = 1;
    buffer(1) = u;
else
    % wenn nicht leer, dann schiebe eins hoch 
    buff2 = buffer; 
    buffer = [u; buff2(1:end-1)];
end

% Output the buffer
y = buffer';

end

== matlab function Trajectory_Tracking_Final/TRajcetory from design reference/Subsystem2/MATLAB Function5 ==
  data: t input; y output; xx input; yy input; t output
function [y, t] = trajectory_s_curve(t,xx,yy)
    total_time = 15;
    t_waypoints = linspace(0, total_time, size(xx, 1));

    waypoints =[xx;yy];

 y = zeros(2,21);

if t < 10
 y(1,:) =  xx(1)*ones(1,21);
  y(2,:) =  yy(1)*ones(1,21);
else
    t = t-10;
    % t = t*5;
    t = mod(t,total_time);
    t_span = [t:0.05:t+(20*0.05)];
for i = 1:21
    y(1,i) =  interp1(t_waypoints, xx, t_span(i), 'spline', 'extrap');
    y(2,i) =  interp1(t_waypoints, yy, t_span(i), 'spline', 'extrap');
    % Function handles for spline interpolation
   % for i = 1:100;
   %     t = i*0.5;
%     x_ref =  interp1(t_waypoints, xx, t, 'spline', 'extrap');
%     y_ref =  interp1(t_waypoints, yy, t, 'spline', 'extrap');
% % scatter(x_ref,y_ref)
% hold on 
%    end
    % y = [x_ref; y_ref];
 
end
end

== matlab function Trajectory_Tracking_Final/TRajcetory from design reference/Subsystem3/MATLAB Function ==
  data: x output; u input; y output
function [x,y]  = fcn(u)

x = u(1);
y = u(2);

== matlab function Trajectory_Tracking_Final/TRajcetory from design reference/Subsystem3/MATLAB Function6 ==
  data: x input; Payload_x output; Payload_y output; Payload_x_der output; Payload_y_der output
function [Payload_x,Payload_y,Payload_x_der,Payload_y_der] = PAyload_calc(x)
Payload_x = x(1)+ 0.5478*x(4);
 Payload_y = x(2)+ 0.5478*x(5);
 Payload_x_der = x(6)+ 0.5478*x(9);
 Payload_y_der = x(7)+ 0.5478*x(10);

== matlab function Trajectory_Tracking_Final/TRajcetory from design reference/Subsystem3/MATLAB Function7 ==
  data: traj input; first_elemt_traj output
function first_elemt_traj = getfirstelement(traj)

first_elemt_traj = traj(:,1);

== matlab function Trajectory_Tracking_Final/TRajcetory from design reference1/Subsystem2/MATLAB Function5 ==
  data: t input; y output; xx input; yy input; t output
function [y, t] = trajectory_s_curve(t,xx,yy)
    total_time = 15;
    t_waypoints = linspace(0, total_time, size(xx, 1));

    waypoints =[xx;yy];

 y = zeros(2,21);

if t < 10
 y(1,:) =  xx(1)*ones(1,21);
  y(2,:) =  yy(1)*ones(1,21);
else
    t = t-10;
    % t = t*5;
    t = mod(t,total_time);
    t_span = [t:0.05:t+(20*0.05)];
for i = 1:21
    y(1,i) =  interp1(t_waypoints, xx, t_span(i), 'spline', 'extrap');
    y(2,i) =  interp1(t_waypoints, yy, t_span(i), 'spline', 'extrap');
    % Function handles for spline interpolation
   % for i = 1:100;
   %     t = i*0.5;
%     x_ref =  interp1(t_waypoints, xx, t, 'spline', 'extrap');
%     y_ref =  interp1(t_waypoints, yy, t, 'spline', 'extrap');
% % scatter(x_ref,y_ref)
% hold on 
%    end
    % y = [x_ref; y_ref];
 
end
end

== matlab function Trajectory_Tracking_Final/TRajcetory from design reference1/Subsystem3/MATLAB Function ==
  data: x output; u input; y output
function [x,y]  = fcn(u)

x = u(1);
y = u(2);

== matlab function Trajectory_Tracking_Final/TRajcetory from design reference1/Subsystem3/MATLAB Function6 ==
  data: x input; Payload_x output; Payload_y output; Payload_x_der output; Payload_y_der output
function [Payload_x,Payload_y,Payload_x_der,Payload_y_der] = PAyload_calc(x)
Payload_x = x(1)+ 0.5478*x(4);
 Payload_y = x(2)+ 0.5478*x(5);
 Payload_x_der = x(6)+ 0.5478*x(9);
 Payload_y_der = x(7)+ 0.5478*x(10);

== matlab function Trajectory_Tracking_Final/TRajcetory from design reference1/Subsystem3/MATLAB Function7 ==
  data: traj input; first_elemt_traj output
function first_elemt_traj = getfirstelement(traj)

first_elemt_traj = traj(:,1);

== matlab function Trajectory_Tracking_Final/TRajcetory from design reference1/Subsystem5/Delete L ==
  data: x10 input; x_8 output
function x_8 = fcn(x10)
relevantstates = [1,2,4,5,6,7,9,10];
x_8 =x10(relevantstates);

== matlab function Trajectory_Tracking_Final/TRajcetory from design reference1/Subsystem5/MATLAB Function ==
  data: x input; x_warm output
function x_warm = fcn(x)
x_warm = [x(:,3:end) x(:,end)];

== matlab function Trajectory_Tracking_Final/Subsystem1/Subsystem/Subsystem5/Subsystem10/MATLAB Function11 ==
  settings: updateMethod=DISCRETE
  data: u input; y output size=[1,N_Coeff]; Initial_Buffer input
function y = CircularBuffer(u,Initial_Buffer)
%#codegen
% Function to implement a simple N element circular buffer

% Define the internal buffer variable as persistent
persistent buffer



% Initialize the buffer the first time through
if isempty(buffer)
    % Initialize the buffer
    buffer = Initial_Buffer*u;
    % buff_entrys = 1;
    buffer(1) = u;
else
    % wenn nicht leer, dann schiebe eins hoch 
    buff2 = buffer; 
    buffer = [u; buff2(1:end-1)];
end

% Output the buffer
y = buffer';

end

== matlab function Trajectory_Tracking_Final/TRajcetory from design reference1/Subsystem5/MATLAB Function1 ==
  data: lam_g input; lam_g_warm output
function lam_g_warm = fcn(lam_g)
lam_g_warm = lam_g;

== matlab function Trajectory_Tracking_Final/TRajcetory from design reference1/Subsystem5/MATLAB Function10 ==
  data: x_18 input; x_out output; x_9 input
function x_out = add_int(x_18,x_9)
x_out = zeros(10,1);
x_out(1) = x_18(1);
x_out(2) = x_18(2);
x_out(3) = x_18(3);
x_out(4) = x_18(4);
x_out(5) = x_18(5);
x_out(6) = x_18(6);
x_out(7) = x_18(7);
x_out(8) = x_18(8);
x_out(9) = x_9(9);
x_out(10) = x_9(10);
% x_out(11) = x_9(11);
% x_out(12) = x_9(12);

if x_out(1) < 0 
    x_out(1) = 0;
end
if x_out(2) < 0 
    x_out(2) = 0;
end

== matlab function Trajectory_Tracking_Final/TRajcetory from design reference1/Subsystem5/MATLAB Function2 ==
  data: u input; u_warm output size=DimU; Delay input
function u_warm = fcn(u,Delay)
Delay = 3;
u_warm = [u(:,(Delay+1):end) u(:,end)];

== matlab function Trajectory_Tracking_Final/TRajcetory from design reference1/Subsystem5/MATLAB Function3 ==
  data: u input; u_new output size=[2,Delay]; u_plant output size=[2,1]; x input; x_new output; Delay input
function [u_new,u_plant,x_new] = fcn(u,x,Delay)
% size(u)
% size(x)
Delay = 3;
u_new = zeros(2,Delay);
u_new = u(:,1:Delay);
x_new = x(:,2);
u_plant = u(:,Delay+1);

== matlab function Trajectory_Tracking_Final/TRajcetory from design reference1/Subsystem5/Subsystem4/MATLAB Function8 ==
  data: traj input; first_elemt_traj output
function first_elemt_traj = getfirstelement(traj)

first_elemt_traj = traj(:,1);

== matlab function Trajectory_Tracking_Final/TRajcetory from design reference/MATLAB Function ==
  data: u input; y output
function y = fcn(u)

y = u(1:2,:);

== matlab function Trajectory_Tracking_Final/Subsystem1/Subsystem/Subsystem5/Subsystem11/MATLAB Function11 ==
  settings: updateMethod=DISCRETE
  data: u input; y output size=[1,N_Coeff]; Initial_Buffer input
function y = CircularBuffer(u,Initial_Buffer)
%#codegen
% Function to implement a simple N element circular buffer

% Define the internal buffer variable as persistent
persistent buffer



% Initialize the buffer the first time through
if isempty(buffer)
    % Initialize the buffer
    buffer = Initial_Buffer*u;
    % buff_entrys = 1;
    buffer(1) = u;
else
    % wenn nicht leer, dann schiebe eins hoch 
    buff2 = buffer; 
    buffer = [u; buff2(1:end-1)];
end

% Output the buffer
y = buffer';

end

== matlab function Trajectory_Tracking_Final/Subsystem1/Subsystem/Subsystem5/Subsystem12/MATLAB Function11 ==
  settings: updateMethod=DISCRETE
  data: u input; y output size=[1,N_Coeff]; Initial_Buffer input
function y = CircularBuffer(u,Initial_Buffer)
%#codegen
% Function to implement a simple N element circular buffer

% Define the internal buffer variable as persistent
persistent buffer



% Initialize the buffer the first time through
if isempty(buffer)
    % Initialize the buffer
    buffer = Initial_Buffer*u;
    % buff_entrys = 1;
    buffer(1) = u;
else
    % wenn nicht leer, dann schiebe eins hoch 
    buff2 = buffer; 
    buffer = [u; buff2(1:end-1)];
end

% Output the buffer
y = buffer';

end

== matlab function Trajectory_Tracking_Final/Subsystem1/Subsystem/Subsystem5/Subsystem13/MATLAB Function11 ==
  settings: updateMethod=DISCRETE
  data: u input; y output size=[1,N_Coeff]; Initial_Buffer input
function y = CircularBuffer(u,Initial_Buffer)
%#codegen
% Function to implement a simple N element circular buffer

% Define the internal buffer variable as persistent
persistent buffer



% Initialize the buffer the first time through
if isempty(buffer)
    % Initialize the buffer
    buffer = Initial_Buffer*u;
    % buff_entrys = 1;
    buffer(1) = u;
else
    % wenn nicht leer, dann schiebe eins hoch 
    buff2 = buffer; 
    buffer = [u; buff2(1:end-1)];
end

% Output the buffer
y = buffer';

end

== matlab function Trajectory_Tracking_Final/Subsystem1/Subsystem/Subsystem5/Subsystem14/MATLAB Function11 ==
  settings: updateMethod=DISCRETE
  data: u input; y output size=[1,N_Coeff]; Initial_Buffer input
function y = CircularBuffer(u,Initial_Buffer)
%#codegen
% Function to implement a simple N element circular buffer

% Define the internal buffer variable as persistent
persistent buffer



% Initialize the buffer the first time through
if isempty(buffer)
    % Initialize the buffer
    buffer = Initial_Buffer*u;
    % buff_entrys = 1;
    buffer(1) = u;
else
    % wenn nicht leer, dann schiebe eins hoch 
    buff2 = buffer; 
    buffer = [u; buff2(1:end-1)];
end

% Output the buffer
y = buffer';

end
